simulink model "test_Dynamics_coupled_MandC"  (R2021b)
settings: Solver=ode4  StartTime=0.0  StopTime=0.01  FixedStep=0.01  RelTol=1e-3  EnableMultiTasking=on
InitFcn:
  | % ************** Initiate forces
  | % f0=[0;0;0;0;0;0];
  | % f0=[0;0;0;0;0;0;0];
  | %f_0=[0;0;0];
  | f_m=[0;1];
  | f_e=[0;0;0;0;0;0];
  | % ************** Initiate states
  | q_m=[0;0];
  | %q_dot_m=[0;0];
  | P=[0;0;0];
  | V_I0=[0;0;0];
  | % ************** Load main
  | %run(Main.m)
StopFcn:
  | format long
  | qddot=out.qddot.data(:,1)
  | qddot_ref=out.qddot_ref.data(1,:)
values from neighbouring files (symbols this model uses):
  diag_M = diagonalize(M_frak0, M_frak)    [Create_Robot.m]    (also in Main.m; diagonalize.m = zeros(6*(n+1),6*(n+1)); test_C_Main.m)
  f_0 = [0;0;0]    [Create_Robot.m]    (also in Main.m = [0;0;0;0;0;0]; test_C_Main.m)
  I0 = eye(3)*416.667    [Create_Robot.m]    (also in Main.m; test_C_Main.m)
  iota0 = [1 0 0; 0 1 0;zeros(3,3);0 0 1]    [Create_Robot.m]    (also in Main.m = eye(6,6); test_C_Main.m)
  m0 = 100    [Create_Robot.m]    (also in Main.m = 10; test_C_Main.m)
  mm = [2 2]    [Create_Robot.m]    (also in Main.m; test_C_Main.m)
  out = sim('test_Dynamics_coupled_full',0.01)    [Main.m]
  q_dot_m = [0;0]    [Create_Robot.m]    (also in Main.m; test_C_Main.m)
  X = [0 -x(3) x(2) ; x(3) 0 -x(1) ; -x(2) x(1) 0 ]    [skewsym.m]
  Xi_m_matrix = zeros(6*n,n)    [Create_Robot.m]    (also in Main.m; test_C_Main.m)
undefined symbols (not defined in the file or in its folder): Xi_m, Y, Z
libraries: sm_lib x11, nesl_utility x9
(part 1 of 2)
settings Model: Creator=Bmmog  LastModifiedBy=Bmmog
settings SimscapeCC: SimscapeLogType=all  SimscapeLogSimulationStatistics=on

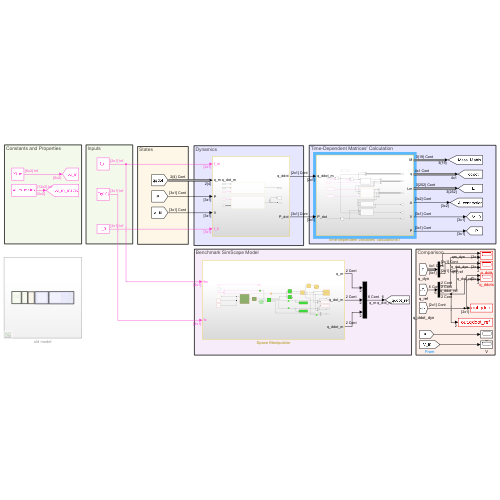
[thumbnail: Simulink's stored preview of the top-level diagram]
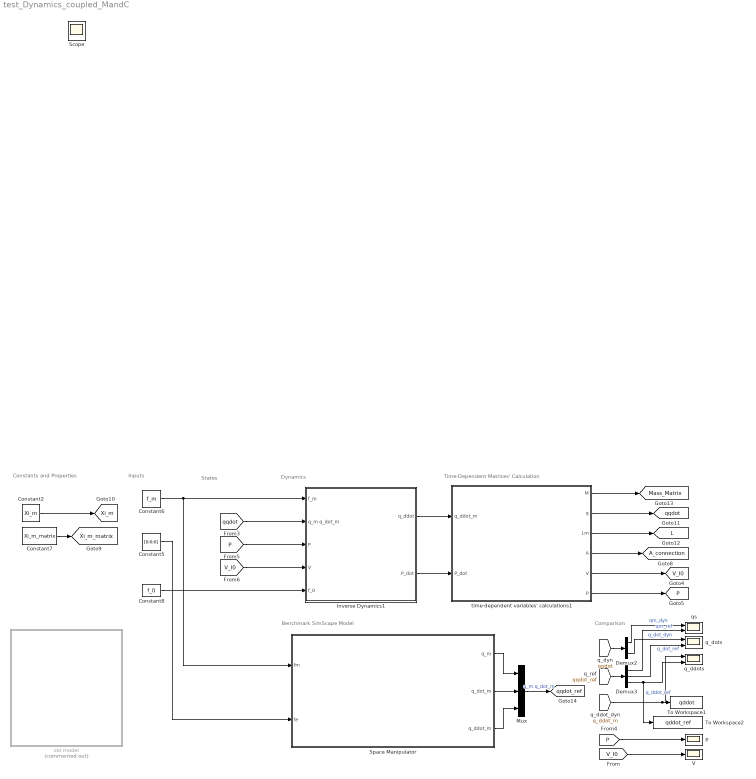
== system test_Dynamics_coupled_MandC ==
  note: States
  note: Constants and Properties
  note: Benchmark SimScape Model
  note: Comparison
  note: Inputs
  note: Dynamics
  note: Time-Dependent Matrices' Calculation
  Constant2 : Constant  Value=Xi_m  VectorParams1D=off
  Constant5 : Constant  Value=[0;0;0]  VectorParams1D=off
  Constant6 : Constant  Value=f_m  VectorParams1D=off
  Constant7 : Constant  Value=Xi_m_matrix  VectorParams1D=off
  Constant8 : Constant  Value=f_0  VectorParams1D=off
  Demux2 : Demux  Outputs=2
  Demux3 : Demux  Outputs=3
  Inverse Dynamics1 : Subsystem
  Mux : Mux  Inputs=3
  P : Scope
  Space Manipulator : Subsystem
  To Workspace1 : ToWorkspace  VariableName=qddot  SaveFormat=Timeseries  SampleTime=-1
  To Workspace2 : ToWorkspace  VariableName=qddot_ref  SaveFormat=Timeseries  SampleTime=-1
  V : Scope
  old model : Subsystem  Commented=on
  q_ddots : Scope  NumInputPorts=2
  q_dots : Scope  NumInputPorts=2
  qs : Scope  NumInputPorts=2
  time-dependent variables' calculations1 : Subsystem
  Scope : Scope
  tag scope: A_connection=global, L=global, Mass_Matrix=global, P=global, V_I0=global, Xi_m=global, Xi_m_matrix=global, qqdot=global, qqdot_ref=global
  wires:
  [V_I0] -> Inverse Dynamics1/4(V)
  Demux2/2 -> q_dots/1  "q_dot_dyn"
  Mux/1 -> [qqdot_ref]  "q_m q_dot_m"
  Space Manipulator/1(q_m) -> Mux/1
  [qqdot] -> Inverse Dynamics1/2(q_m q_dot_m)
  [q_ddot_m] -> q_ddots/1, To Workspace1/1
  Space Manipulator/2(q_dot_m) -> Mux/2
  Constant6/1 -> Space Manipulator/1(fm), Inverse Dynamics1/1(f_m)
  time-dependent variables' calculations1/1(M) -> [Mass_Matrix]
  Constant2/1 -> [Xi_m]
  [qqdot_ref] -> Demux3/1
  Demux3/1 -> qs/2  "qm_ref"
  [qqdot] -> Demux2/1
  Inverse Dynamics1/1(q_ddot) -> time-dependent variables' calculations1/1(q_ddot_m)
  Demux2/1 -> qs/1  "qm_dyn"
  Constant7/1 -> [Xi_m_matrix]
  Constant5/1 -> Space Manipulator/2(fe)
  Demux3/2 -> q_dots/2  "q_dot_ref"
  time-dependent variables' calculations1/2(q) -> [qqdot]
  Space Manipulator/3(q_ddot_m) -> Mux/3
  [P] -> Inverse Dynamics1/3(P)
  Constant8/1 -> Inverse Dynamics1/5(f_0)
  time-dependent variables' calculations1/6(P) -> [P]
  Inverse Dynamics1/2(P_dot) -> time-dependent variables' calculations1/2(P_dot)
  time-dependent variables' calculations1/3(Lm) -> [L]
  Demux3/3 -> To Workspace2/1, q_ddots/2  "q_ddot_ref"
  time-dependent variables' calculations1/5(V) -> [V_I0]
  time-dependent variables' calculations1/4(A) -> [A_connection]
  [P] -> P/1
  [V_I0] -> V/1

== system test_Dynamics_coupled_MandC/Inverse Dynamics1 ==
  f_m : Inport
  q_m q_dot_m : Inport  Port=2
  P : Inport  Port=3
  V : Inport  Port=4
  f_0 : Inport  Port=5
  Euler Poincare : Subsystem
  Internal Dynamics : Subsystem
  q_ddot : Outport
  P_dot : Outport  Port=2
  tag scope: q_ddot_m=global
  wires:
  f_m/1 -> Internal Dynamics/1(f_m)
  q_m q_dot_m/1 -> Internal Dynamics/2(q_m q_dot_m)
  Internal Dynamics/1(q_ddot) -> [q_ddot_m], q_ddot/1  "q_ddot"
  Euler Poincare/1(P_dot) -> P_dot/1  "P_dot"
  f_0/1 -> Euler Poincare/3(f_0)
  P/1 -> Euler Poincare/1(P)
  V/1 -> Euler Poincare/2(V)

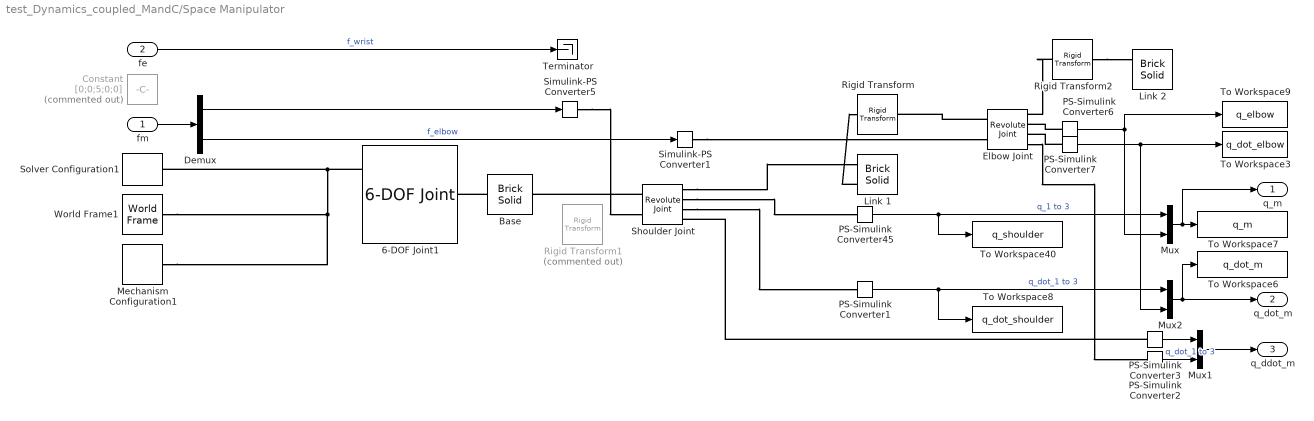
== system test_Dynamics_coupled_MandC/Space Manipulator ==
  fm : Inport
  fe : Inport  Port=2
  6-DOF Joint1 : sm_lib/Joints/6-DOF Joint  JointMode=Normal  SenseConstraintForce=off  SenseConstraintForceX=off  SenseConstraintForceY=off  SenseConstraintForceZ=off  SenseConstraintTorque=off  SenseConstraintTorqueX=off  SenseConstraintTorqueY=off  SenseConstraintTorqueZ=off  SenseTotalForce=off  SenseTotalForceX=off  SenseTotalForceY=off  SenseTotalForceZ=off  SenseTotalTorque=off  SenseTotalTorqueX=off  SenseTotalTorqueY=off  SenseTotalTorqueZ=off  CompositeWrenchDir=FollowerOnBase  CompositeWrenchFrame=BaseFrame  PxEquilibriumPosition=0  PxEquilibriumPositionUnits=m  PxSpringStiffness=0  PxSpringStiffnessUnits=N/m  PxDampingCoefficient=0  PxDampingCoefficientUnits=N/(m/s)  PxTorqueActuationMode=InputTorque  PxMotionActuationMode=ComputedMotion  PxSensePosition=off  PxSenseVelocity=off  PxSenseAcceleration=off  PxSenseTorqueForce=off  PxSenseLowerLimitTorqueForce=off  PxSenseUpperLimitTorqueForce=off  PxLowerLimitSpecify=off  PxLowerLimitBound=-1  PxLowerLimitBoundUnits=m  PxLowerLimitStiffness=1e6  PxLowerLimitStiffnessUnits=N/m  PxLowerLimitDamping=1e3  PxLowerLimitDampingUnits=N/(m/s)  PxLowerLimitTransitionRegionWidth=1e-4  PxLowerLimitTransitionRegionWidthUnits=m  PxUpperLimitSpecify=off  PxUpperLimitBound=1  PxUpperLimitBoundUnits=m  PxUpperLimitStiffness=1e6  PxUpperLimitStiffnessUnits=N/m  PxUpperLimitDamping=1e3  PxUpperLimitDampingUnits=N/(m/s)  PxUpperLimitTransitionRegionWidth=1e-4  PxUpperLimitTransitionRegionWidthUnits=m  PxPositionTargetSpecify=on  PxPositionTargetPriority=High  PxPositionTargetValue=0  PxPositionTargetValueUnits=m  PxVelocityTargetSpecify=off  PxVelocityTargetPriority=High  PxVelocityTargetValue=0  PxVelocityTargetValueUnits=m/s  PyEquilibriumPosition=0  PyEquilibriumPositionUnits=m  PySpringStiffness=0  PySpringStiffnessUnits=N/m  PyDampingCoefficient=0  PyDampingCoefficientUnits=N/(m/s)  PyTorqueActuationMode=NoTorque  PyMotionActuationMode=ComputedMotion  PySensePosition=off  PySenseVelocity=off  PySenseAcceleration=off  PySenseTorqueForce=off  PySenseLowerLimitTorqueForce=off  PySenseUpperLimitTorqueForce=off  PyLowerLimitSpecify=off  PyLowerLimitBound=-1  PyLowerLimitBoundUnits=m  PyLowerLimitStiffness=1e6  PyLowerLimitStiffnessUnits=N/m  PyLowerLimitDamping=1e3  PyLowerLimitDampingUnits=N/(m/s)  PyLowerLimitTransitionRegionWidth=1e-4  PyLowerLimitTransitionRegionWidthUnits=m  PyUpperLimitSpecify=off  PyUpperLimitBound=1  PyUpperLimitBoundUnits=m  PyUpperLimitStiffness=1e6  PyUpperLimitStiffnessUnits=N/m  PyUpperLimitDamping=1e3  PyUpperLimitDampingUnits=N/(m/s)  PyUpperLimitTransitionRegionWidth=1e-4  PyUpperLimitTransitionRegionWidthUnits=m  PyPositionTargetSpecify=on  PyPositionTargetPriority=High  PyPositionTargetValue=0  PyPositionTargetValueUnits=m  PyVelocityTargetSpecify=off  PyVelocityTargetPriority=High  PyVelocityTargetValue=0  PyVelocityTargetValueUnits=m/s  PzEquilibriumPosition=0  PzEquilibriumPositionUnits=m  PzSpringStiffness=0  PzSpringStiffnessUnits=N/m  PzDampingCoefficient=0  PzDampingCoefficientUnits=N/(m/s)  PzTorqueActuationMode=NoTorque  PzMotionActuationMode=ComputedMotion  PzSensePosition=off  PzSenseVelocity=off  PzSenseAcceleration=off  PzSenseTorqueForce=off  PzSenseLowerLimitTorqueForce=off  PzSenseUpperLimitTorqueForce=off  PzLowerLimitSpecify=off  PzLowerLimitBound=-1  PzLowerLimitBoundUnits=m  PzLowerLimitStiffness=1e6  PzLowerLimitStiffnessUnits=N/m  PzLowerLimitDamping=1e3  PzLowerLimitDampingUnits=N/(m/s)  PzLowerLimitTransitionRegionWidth=1e-4  PzLowerLimitTransitionRegionWidthUnits=m  PzUpperLimitSpecify=off  PzUpperLimitBound=1  PzUpperLimitBoundUnits=m  PzUpperLimitStiffness=1e6  PzUpperLimitStiffnessUnits=N/m  PzUpperLimitDamping=1e3  PzUpperLimitDampingUnits=N/(m/s)  PzUpperLimitTransitionRegionWidth=1e-4  PzUpperLimitTransitionRegionWidthUnits=m  PzPositionTargetSpecify=on  PzPositionTargetPriority=High  PzPositionTargetValue=0  PzPositionTargetValueUnits=m  PzVelocityTargetSpecify=off  PzVelocityTargetPriority=High  PzVelocityTargetValue=0  PzVelocityTargetValueUnits=m/s  SphDefPosRotationMethod=None  SphDefPosRotationAngleUnits=deg  SphDefPosRotationStandardAxis=+Z  SphDefPosRotationAngle=0.0  SphDefPosRotationArbitraryAxis=[0 0 1]  SphDefPosFollAlignAxisA=+X  SphDefPosBaseAlignAxisA=+Y  SphDefPosFollAlignAxisB=+Y  SphDefPosBaseAlignAxisB=+Z  SphDefPosRotationSequenceAxes=FollowerAxes  SphDefPosRotationSequence=XYX  SphDefPosRotationSequenceAngles=[0 0 0]  SphDefPosRotationSequenceAnglesUnits=deg  SphDefPosRotationMatrix=[1 0 0; 0 1 0; 0 0 1]  SphEqPosRotationMethod=None  SphEqPosRotationAngleUnits=deg  SphEqPosRotationStandardAxis=+Z  SphEqPosRotationAngle=0.0  SphEqPosRotationArbitraryAxis=[0 0 1]  SphEqPosFollAlignAxisA=+X  SphEqPosBaseAlignAxisA=+Y  SphEqPosFollAlignAxisB=+Y  SphEqPosBaseAlignAxisB=+Z  SphEqPosRotationSequenceAxes=FollowerAxes  SphEqPosRotationSequence=XYX  SphEqPosRotationSequenceAngles=[0 0 0]  SphEqPosRotationSequenceAnglesUnits=deg  SphEqPosRotationMatrix=[1 0 0; 0 1 0; 0 0 1]  SphSpringStiffness=0  SphSpringStiffnessUnits=N*m/deg  SphDampingCoefficient=0  SphDampingCoefficientUnits=N*m/(deg/s)  SphActuateTorqueX=off  SphActuateTorqueY=off  SphActuateTorqueZ=off  SphActuateTorque=off  SphTorqueActuationMode=NoTorque  SphMotionActuationMode=ComputedMotion  SphActuationFrame=BaseFrame  SphSensePosition=off  SphSenseVelocityX=off  SphSenseVelocityY=off  SphSenseVelocityZ=off  SphSenseVelocity=off  SphSenseAccelerationX=off  SphSenseAccelerationY=off  SphSenseAccelerationZ=off  SphSenseAcceleration=off  SphSenseTorqueX=off  SphSenseTorqueY=off  SphSenseTorqueZ=off  SphSenseTorqueForce=off  SphSenseLowerLimitTorqueMag=off  SphSenseUpperLimitTorqueMag=off  SphSensingFrame=BaseFrame  SphLowerLimitSpecify=off  SphLowerLimitBound=15  SphLowerLimitBoundUnits=deg  SphLowerLimitStiffness=1e4  SphLowerLimitStiffnessUnits=N*m/deg  SphLowerLimitDamping=10  SphLowerLimitDampingUnits=N*m/(deg/s)  SphLowerLimitTransitionRegionWidth=0.1  SphLowerLimitTransitionRegionWidthUnits=deg  SphUpperLimitSpecify=off  SphUpperLimitBound=45  SphUpperLimitBoundUnits=deg  SphUpperLimitStiffness=1e4  SphUpperLimitStiffnessUnits=N*m/deg  SphUpperLimitDamping=10  SphUpperLimitDampingUnits=N*m/(deg/s)  SphUpperLimitTransitionRegionWidth=0.1  SphUpperLimitTransitionRegionWidthUnits=deg  SphPositionTargetRotationMethod=RotationSequence  SphPositionTargetRotationAngleUnits=deg  SphPositionTargetRotationStandardAxis=+Z  SphPositionTargetRotationAngle=0.0  SphPositionTargetRotationArbitraryAxis=[0 0 1]  SphPositionTargetFollAlignAxisA=+X  SphPositionTargetBaseAlignAxisA=+Y  SphPositionTargetFollAlignAxisB=+Y  SphPositionTargetBaseAlignAxisB=+Z  SphPositionTargetRotationSequenceAxes=FollowerAxes  SphPositionTargetRotationSequence=ZYX  SphPositionTargetRotationSequenceAngles=[0 0 0]  SphPositionTargetRotationSequenceAnglesUnits=deg  SphPositionTargetRotationMatrix=[1 0 0; 0 1 0; 0 0 1]  SphPositionTargetSpecify=off  SphPositionTargetPriority=High  SphVelocityTargetValue=[0 0.5 0.5]  SphVelocityTargetValueUnits=rad/s  SphVelocityTargetSpecify=off  SphVelocityTargetPriority=High  SphVelocityTargetInFollowerFrame=on
  Base : sm_lib/Body Elements/Brick Solid  GraphicAmbientColor=[0.15 0.15 0.15 1.0]  BasedOnType=Mass  BrickDimensions=[5, 5, 5]  BrickDimensionUnits=m  CenterOfMass=[0 0 0]  CenterOfMassUnits=m  GraphicDiffuseColor=[0.5 0.5 0.5]  Density=1000  DensityUnits=kg/m^3  DoExposeReferenceFrame=on  GraphicEmissiveColor=[0.0 0.0 0.0 1.0]  ExportEntireGeometry=off  SerializedFrames=<Frames><Frame><Id>Frame1</Id><Value><Name>F1</Name><Origin><Source>GeometricFeature</Source><FeatureName>+z surface</FeatureName></Origin><PrimaryAxis><DefinedDirection>+X</DefinedDirection><Source>ReferenceFrame</Source><SourceDirection>+Z</SourceDirection><FeatureName></FeatureName></PrimaryAxis><SecondaryAxis><DefinedDirection>+Z</DefinedDirection><Source>ReferenceFrame</Source><SourceDirection>+X</SourceDirection><FeatureName></FeatureName></SecondaryAxis></Value></Frame></Frames>  MarkerShape=Sphere  MarkerSize=10  GraphicType=FromGeometry  InertiaType=Custom  Mass=m0  MassUnits=kg  MomentsOfInertia=[I0(1,1) I0(2,2) I0(3,3)]  MomentsOfInertiaUnits=kg*m^2  GraphicOpacity=1.0  ProductsOfInertia=[0 0 0]  ProductsOfInertiaUnits=kg*m^2  GraphicShininess=75  GraphicSpecularColor=[0.5 0.5 0.5 1.0]  GraphicVisPropType=SimpleVisualProperties
  Constant : Constant  Commented=on  Value=[0;0;5;0;0]
  Demux : Demux  Outputs=2
  Elbow Joint : sm_lib/Joints/Revolute Joint  JointMode=Normal  SenseConstraintForce=off  SenseConstraintForceX=off  SenseConstraintForceY=off  SenseConstraintForceZ=off  SenseConstraintTorque=off  SenseConstraintTorqueX=off  SenseConstraintTorqueY=off  SenseConstraintTorqueZ=off  SenseTotalForce=off  SenseTotalForceX=off  SenseTotalForceY=off  SenseTotalForceZ=off  SenseTotalTorque=off  SenseTotalTorqueX=off  SenseTotalTorqueY=off  SenseTotalTorqueZ=off  CompositeWrenchDir=FollowerOnBase  CompositeWrenchFrame=BaseFrame  EquilibriumPosition=0  EquilibriumPositionUnits=rad  SpringStiffness=0  SpringStiffnessUnits=N*m/rad  DampingCoefficient=0  DampingCoefficientUnits=N*m/(rad/s)  TorqueActuationMode=InputTorque  MotionActuationMode=ComputedMotion  SensePosition=on  SenseVelocity=on  SenseAcceleration=on  SenseTorqueForce=off  SenseLowerLimitTorqueForce=off  SenseUpperLimitTorqueForce=off  LowerLimitSpecify=off  LowerLimitBound=-90  LowerLimitBoundUnits=deg  LowerLimitStiffness=1e4  LowerLimitStiffnessUnits=N*m/deg  LowerLimitDamping=10  LowerLimitDampingUnits=N*m/(deg/s)  LowerLimitTransitionRegionWidth=0.1  LowerLimitTransitionRegionWidthUnits=deg  UpperLimitSpecify=off  UpperLimitBound=90  UpperLimitBoundUnits=deg  UpperLimitStiffness=1e4  UpperLimitStiffnessUnits=N*m/deg  UpperLimitDamping=10  UpperLimitDampingUnits=N*m/(deg/s)  UpperLimitTransitionRegionWidth=0.1  UpperLimitTransitionRegionWidthUnits=deg  PositionTargetSpecify=on  PositionTargetPriority=High  PositionTargetValue=q_m(2)  PositionTargetValueUnits=rad  VelocityTargetSpecify=on  VelocityTargetPriority=High  VelocityTargetValue=q_dot_m(2)  VelocityTargetValueUnits=rad/s
  "Link 1 " : sm_lib/Body Elements/Brick Solid  GraphicAmbientColor=[0.15 0.15 0.15 1.0]  BasedOnType=Mass  BrickDimensions=[0.1, 0.1, 4.5]  BrickDimensionUnits=m  CenterOfMass=[0 0 0]  CenterOfMassUnits=m  GraphicDiffuseColor=[0.5 0.5 0.5]  Density=1000  DensityUnits=kg/m^3  DoExposeReferenceFrame=on  GraphicEmissiveColor=[0.0 0.0 0.0 1.0]  ExportEntireGeometry=off  SerializedFrames=<Frames><Frame><Id>Frame1</Id><Value><Name>F1</Name><Origin><Source>GeometricFeature</Source><FeatureName>-z surface</FeatureName></Origin><PrimaryAxis><DefinedDirection>+X</DefinedDirection><Source>ReferenceFrame</Source><SourceDirection>+Z</SourceDirection><FeatureName></FeatureName></PrimaryAxis><SecondaryAxis><DefinedDirection>+Z</DefinedDirection><Source>ReferenceFrame</Source><SourceDirection>+X</SourceDirection><FeatureName></FeatureName></SecondaryAxis></Value></Frame><Frame><Id>Frame2</Id><Value><Name>F2</Name><Origin><Source>GeometricFeature</Source><FeatureName>+z surface</FeatureName></Origin><PrimaryAxis><DefinedDirection>+X</DefinedDirection><Source>ReferenceFrame</Source><SourceDirection>+Z</SourceDirection><FeatureName></FeatureName></PrimaryAxis><SecondaryAxis><DefinedDirection>+Z</DefinedDirection><Source>ReferenceFrame</Source><SourceDirection>+X</SourceDirection><FeatureName></FeatureName></SecondaryAxis></Value></Frame></Frames>  MarkerShape=Sphere  MarkerSize=10  GraphicType=FromGeometry  InertiaType=Custom  Mass=mm(1)  MassUnits=kg  MomentsOfInertia=[3.37667 3.37667 0.00333333]  MomentsOfInertiaUnits=kg*m^2  GraphicOpacity=1.0  ProductsOfInertia=[0 0 0]  ProductsOfInertiaUnits=kg*m^2  GraphicShininess=75  GraphicSpecularColor=[0.5 0.5 0.5 1.0]  GraphicVisPropType=SimpleVisualProperties
  Link 2 : sm_lib/Body Elements/Brick Solid  GraphicAmbientColor=[0.15 0.15 0.15 1.0]  BasedOnType=Mass  BrickDimensions=[0.1, 0.1,4.5]  BrickDimensionUnits=m  CenterOfMass=[0 0 0]  CenterOfMassUnits=m  GraphicDiffuseColor=[0.5 0.5 0.5]  Density=1000  DensityUnits=kg/m^3  DoExposeReferenceFrame=on  GraphicEmissiveColor=[0.0 0.0 0.0 1.0]  ExportEntireGeometry=off  SerializedFrames=<Frames><Frame><Id>Frame1</Id><Value><Name>F1</Name><Origin><Source>GeometricFeature</Source><FeatureName>-z surface</FeatureName></Origin><PrimaryAxis><DefinedDirection>+X</DefinedDirection><Source>ReferenceFrame</Source><SourceDirection>+Z</SourceDirection><FeatureName></FeatureName></PrimaryAxis><SecondaryAxis><DefinedDirection>+Z</DefinedDirection><Source>ReferenceFrame</Source><SourceDirection>+Y</SourceDirection><FeatureName></FeatureName></SecondaryAxis></Value></Frame><Frame><Id>Frame2</Id><Value><Name>F2</Name><Origin><Source>GeometricFeature</Source><FeatureName>+z surface</FeatureName></Origin><PrimaryAxis><DefinedDirection>+X</DefinedDirection><Source>ReferenceFrame</Source><SourceDirection>+Z</SourceDirection><FeatureName></FeatureName></PrimaryAxis><SecondaryAxis><DefinedDirection>+Z</DefinedDirection><Source>ReferenceFrame</Source><SourceDirection>+Y</SourceDirection><FeatureName></FeatureName></SecondaryAxis></Value></Frame></Frames>  MarkerShape=Sphere  MarkerSize=10  GraphicType=FromGeometry  InertiaType=Custom  Mass=mm(2)  MassUnits=kg  MomentsOfInertia=[3.37667 3.37667 0.00333333]  MomentsOfInertiaUnits=kg*m^2  GraphicOpacity=1.0  ProductsOfInertia=[0 0 0]  ProductsOfInertiaUnits=kg*m^2  GraphicShininess=75  GraphicSpecularColor=[0.5 0.5 0.5 1.0]  GraphicVisPropType=SimpleVisualProperties
  Mechanism Configuration1 : sm_lib/Utilities/Mechanism Configuration  UniformGravity=Constant  GravityVector=[0 0 0]  GravityUnits=m/s^2  LinearizationDelta=0.001  JointModeTransitionNonlinearIterations=2
  Mux : Mux  Inputs=2
  Mux1 : Mux  Inputs=2
  Mux2 : Mux  Inputs=2
  PS-Simulink Converter{1..3,6..7,45} (6 alike) : nesl_utility/PS-Simulink Converter  PhysicalDomain=network_engine_domain  SubClassName=ps_output  LeftPortType=input  RightPortType=output  PseudoPeriodic=off  Frequencies=[]  Unit=inherit  AffineConversion=off
      settings: SourceProductBaseCode=PW,SS
  Rigid Transform : sm_lib/Frames and Transforms/Rigid Transform  TranslationMethod=None  TranslationStandardOffset=0  TranslationLengthUnit=m  TranslationStandardAxis=+Z  TranslationCartesianOffset=[0 0 0]  TranslationROffset=0  TranslationROffsetUnits=m  TranslationZOffset=0  TranslationZOffsetUnits=m  TranslationThetaOffset=0  TranslationThetaOffsetUnits=deg  RotationMethod=StandardAxis  RotationAngleUnits=deg  RotationStandardAxis=+X  RotationAngle=90  RotationArbitraryAxis=[0 0 1]  FollAlignAxisA=+X  BaseAlignAxisA=+Y  FollAlignAxisB=+Y  BaseAlignAxisB=+Z  RotationSequenceAxes=FollowerAxes  RotationSequence=XYX  RotationSequenceAngles=[0 0 0]  RotationSequenceAnglesUnits=deg  RotationMatrix=[1 0 0; 0 1 0; 0 0 1]
  Rigid Transform1 : sm_lib/Frames and Transforms/Rigid Transform  Commented=on  TranslationMethod=Cartesian  TranslationStandardOffset=0  TranslationLengthUnit=m  TranslationStandardAxis=+Z  TranslationCartesianOffset=[0 0 2.5]  TranslationROffset=0  TranslationROffsetUnits=m  TranslationZOffset=0  TranslationZOffsetUnits=m  TranslationThetaOffset=0  TranslationThetaOffsetUnits=deg  RotationMethod=RotationMatrix  RotationAngleUnits=deg  RotationStandardAxis=+X  RotationAngle=90  RotationArbitraryAxis=[0 0 1]  FollAlignAxisA=+X  BaseAlignAxisA=+Y  FollAlignAxisB=+Y  BaseAlignAxisB=+Z  RotationSequenceAxes=FollowerAxes  RotationSequence=XYX  RotationSequenceAngles=[0 0 0]  RotationSequenceAnglesUnits=deg  RotationMatrix=[0 0 1; 0 -1 0; 1 0 0]
  Rigid Transform2 : sm_lib/Frames and Transforms/Rigid Transform  TranslationMethod=None  TranslationStandardOffset=0  TranslationLengthUnit=m  TranslationStandardAxis=+Z  TranslationCartesianOffset=[0 0 0]  TranslationROffset=0  TranslationROffsetUnits=m  TranslationZOffset=0  TranslationZOffsetUnits=m  TranslationThetaOffset=0  TranslationThetaOffsetUnits=deg  RotationMethod=None  RotationAngleUnits=deg  RotationStandardAxis=+Y  RotationAngle=0  RotationArbitraryAxis=[0 0 1]  FollAlignAxisA=+X  BaseAlignAxisA=+Y  FollAlignAxisB=+Y  BaseAlignAxisB=+Z  RotationSequenceAxes=FollowerAxes  RotationSequence=XYX  RotationSequenceAngles=[0 0 0]  RotationSequenceAnglesUnits=deg  RotationMatrix=[1 0 0; 0 1 0; 0 0 1]
  Shoulder Joint : sm_lib/Joints/Revolute Joint  JointMode=Normal  SenseConstraintForce=off  SenseConstraintForceX=off  SenseConstraintForceY=off  SenseConstraintForceZ=off  SenseConstraintTorque=off  SenseConstraintTorqueX=off  SenseConstraintTorqueY=off  SenseConstraintTorqueZ=off  SenseTotalForce=off  SenseTotalForceX=off  SenseTotalForceY=off  SenseTotalForceZ=off  SenseTotalTorque=off  SenseTotalTorqueX=off  SenseTotalTorqueY=off  SenseTotalTorqueZ=off  CompositeWrenchDir=FollowerOnBase  CompositeWrenchFrame=BaseFrame  EquilibriumPosition=0  EquilibriumPositionUnits=rad  SpringStiffness=0  SpringStiffnessUnits=N*m/rad  DampingCoefficient=0  DampingCoefficientUnits=N*m/(rad/s)  TorqueActuationMode=InputTorque  MotionActuationMode=ComputedMotion  SensePosition=on  SenseVelocity=on  SenseAcceleration=on  SenseTorqueForce=off  SenseLowerLimitTorqueForce=off  SenseUpperLimitTorqueForce=off  LowerLimitSpecify=off  LowerLimitBound=-90  LowerLimitBoundUnits=deg  LowerLimitStiffness=1e4  LowerLimitStiffnessUnits=N*m/deg  LowerLimitDamping=10  LowerLimitDampingUnits=N*m/(deg/s)  LowerLimitTransitionRegionWidth=0.1  LowerLimitTransitionRegionWidthUnits=deg  UpperLimitSpecify=off  UpperLimitBound=90  UpperLimitBoundUnits=deg  UpperLimitStiffness=1e4  UpperLimitStiffnessUnits=N*m/deg  UpperLimitDamping=10  UpperLimitDampingUnits=N*m/(deg/s)  UpperLimitTransitionRegionWidth=0.1  UpperLimitTransitionRegionWidthUnits=deg  PositionTargetSpecify=on  PositionTargetPriority=High  PositionTargetValue=q_m(1)  PositionTargetValueUnits=rad  VelocityTargetSpecify=on  VelocityTargetPriority=High  VelocityTargetValue=q_dot_m(1)  VelocityTargetValueUnits=rad/s
  Simulink-PS Converter1 : nesl_utility/Simulink-PS Converter  PhysicalDomain=network_engine_domain  SubClassName=ps_input  LeftPortType=input  RightPortType=output  PseudoPeriodic=off  Frequencies=[]  NoiseDistribution=none  NoiseParameters=[]  Unit=1  AffineConversion=off  FilteringAndDerivatives=provide  SimscapeFilterOrder=1  InputFilterTimeConstant=0.001  UdotUserProvided=0
      settings: SourceProductBaseCode=PW,SS
  Simulink-PS Converter5 : nesl_utility/Simulink-PS Converter  PhysicalDomain=network_engine_domain  SubClassName=ps_input  LeftPortType=input  RightPortType=output  PseudoPeriodic=off  Frequencies=[]  NoiseDistribution=none  NoiseParameters=[]  Unit=1  AffineConversion=off  FilteringAndDerivatives=provide  SimscapeFilterOrder=1  InputFilterTimeConstant=0.001  UdotUserProvided=0
      settings: SourceProductBaseCode=PW,SS
  Solver Configuration1 : nesl_utility/Solver Configuration  PhysicalDomain=network_engine_domain  SubClassName=solver  LeftPortType=input  RightPortType=generic  Tones=[]  Harmonics=[]  SimulateNoise=off  Profile=off  UseLocalSampling=off  EnableSwitchedLinearOptims=on  FrequencyDomain=off  UseCCode=off  RelTol=0.001  AbsTol=1e-06  MinStep=1e-09  ToWorkspace=off  RevertToSquareIcSolve=off  NumHomotopyIterations=100  PhasorMode=off  PhasorModeNumHarmonics=1  DoDC=off  ResidualTolerance=1e-09  UseLocalSolver=off  LocalSolverChoice=NE_BACKWARD_EULER_ADVANCER  LocalSolverSampleTime=0.001  DoFixedCost=off  MaxNonlinIter=3  MaxModeIter=2  ComputeImpulses=off  ImpulseIterations=2  LinearAlgebra=Sparse  EquationFormulation=NE_TIME_EF  DelaysMemoryBudget=1024  AutomaticFiltering=on  FilteringTimeConstant=0.001  PartitionStorageMethod=AS_NEEDED  PartitionMemoryBudget=1024  PartitionMethod=FAST
      settings: SourceProductBaseCode=PW,SS
  Terminator : Terminator
  To Workspace3 : ToWorkspace  VariableName=q_dot_elbow  SampleTime=-1
  To Workspace40 : ToWorkspace  VariableName=q_shoulder  SampleTime=-1
  To Workspace6 : ToWorkspace  VariableName=q_dot_m  SampleTime=-1
  To Workspace7 : ToWorkspace  VariableName=q_m  SampleTime=-1
  To Workspace8 : ToWorkspace  VariableName=q_dot_shoulder  SampleTime=-1
  To Workspace9 : ToWorkspace  VariableName=q_elbow  SampleTime=-1
  World Frame1 : sm_lib/Frames and Transforms/World Frame
  q_m : Outport
  q_dot_m : Outport  Port=2
  q_ddot_m : Outport  Port=3
  wires:
  PS-Simulink Converter6/1 -> To Workspace9/1, Mux/2
  fm/1 -> Demux/1
  PS-Simulink Converter7/1 -> Mux2/2, To Workspace3/1
  PS-Simulink Converter45/1 -> Mux/1, To Workspace40/1  "q_1 to 3"
  Mux/1 -> q_m/1, To Workspace7/1
  Mux2/1 -> To Workspace6/1, q_dot_m/1
  Demux/2 -> Simulink-PS Converter1/1  "f_elbow"
  PS-Simulink Converter1/1 -> Mux2/1, To Workspace8/1  "q_dot_1 to 3"
  PS-Simulink Converter2/1 -> Mux1/2  "q_dot_1 to 3"
  PS-Simulink Converter3/1 -> Mux1/1
  Mux1/1 -> q_ddot_m/1
  Demux/1 -> Simulink-PS Converter5/1
  fe/1 -> Terminator/1  "f_wrist"
  connections:
  Rigid Transform2/RConn1 -- Link 2/LConn1
  Shoulder Joint/RConn1 -- "Link 1 "/LConn1
  Shoulder Joint/RConn2 -- PS-Simulink Converter45/LConn1
  Elbow Joint/LConn1 -- Rigid Transform/RConn1
  PS-Simulink Converter6/LConn1 -- Elbow Joint/RConn2
  "Link 1 "/LConn2 -- Rigid Transform/LConn1
  Rigid Transform2/LConn1 -- Elbow Joint/RConn1
  Shoulder Joint/RConn3 -- PS-Simulink Converter1/LConn1
  PS-Simulink Converter7/LConn1 -- Elbow Joint/RConn3
  Solver Configuration1/RConn1 -- Mechanism Configuration1/RConn1 -- World Frame1/RConn1 -- 6-DOF Joint1/LConn1
  Elbow Joint/RConn4 -- PS-Simulink Converter2/LConn1
  PS-Simulink Converter3/LConn1 -- Shoulder Joint/RConn4
  Shoulder Joint/LConn1 -- Base/LConn1
  Simulink-PS Converter1/RConn1 -- Elbow Joint/LConn2
  Simulink-PS Converter5/RConn1 -- Shoulder Joint/LConn2
  Base/RConn1 -- 6-DOF Joint1/RConn1

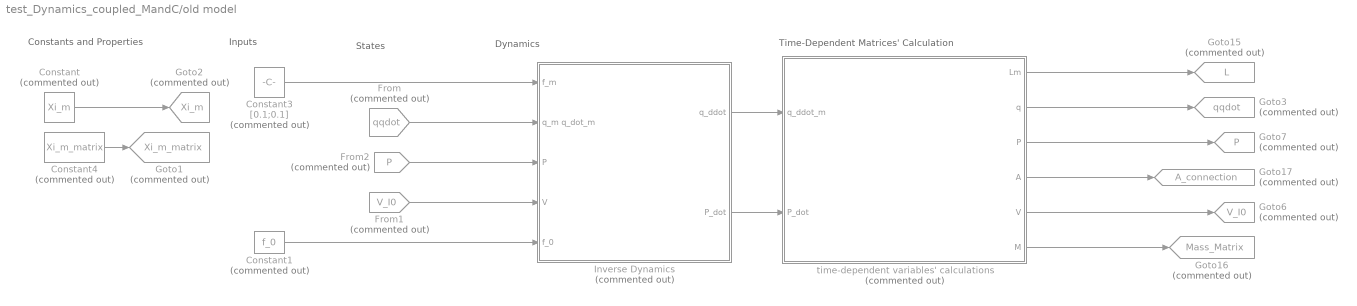
== system test_Dynamics_coupled_MandC/old model ==
  note: States
  note: Inputs
  note: Time-Dependent Matrices' Calculation
  note: Constants and Properties
  note: Dynamics
  Constant : Constant  Commented=on  Value=Xi_m  VectorParams1D=off
  Constant1 : Constant  Commented=on  Value=f_0  VectorParams1D=off
  Constant3 : Constant  Commented=on  Value=[0.1;0.1]  VectorParams1D=off
  Constant4 : Constant  Commented=on  Value=Xi_m_matrix  VectorParams1D=off
  From : From  Commented=on  GotoTag=qqdot  TagVisibility=global
  From1 : From  Commented=on  GotoTag=V_I0  TagVisibility=global
  From2 : From  Commented=on  GotoTag=P  TagVisibility=global
  Goto1 : Goto  Commented=on  GotoTag=Xi_m_matrix  TagVisibility=global
  Goto15 : Goto  Commented=on  GotoTag=L  TagVisibility=global
  Goto16 : Goto  Commented=on  GotoTag=Mass_Matrix  TagVisibility=global
  Goto17 : Goto  Commented=on  GotoTag=A_connection  TagVisibility=global
  Goto2 : Goto  Commented=on  GotoTag=Xi_m  TagVisibility=global
  Goto3 : Goto  Commented=on  GotoTag=qqdot  TagVisibility=global
  Goto6 : Goto  Commented=on  GotoTag=V_I0  TagVisibility=global
  Goto7 : Goto  Commented=on  GotoTag=P  TagVisibility=global
  Inverse Dynamics : Subsystem  Commented=on
  time-dependent variables' calculations : Subsystem  Commented=on
  wires:
  Constant3/1 -> Inverse Dynamics/1(f_m)
  From1/1 -> Inverse Dynamics/4(V)
  time-dependent variables' calculations/6(M) -> Goto16/1
  Inverse Dynamics/2(P_dot) -> time-dependent variables' calculations/2(P_dot)
  time-dependent variables' calculations/2(q) -> Goto3/1
  Constant1/1 -> Inverse Dynamics/5(f_0)
  Constant/1 -> Goto2/1
  time-dependent variables' calculations/1(Lm) -> Goto15/1
  time-dependent variables' calculations/3(P) -> Goto7/1
  From/1 -> Inverse Dynamics/2(q_m q_dot_m)
  Constant4/1 -> Goto1/1
  time-dependent variables' calculations/5(V) -> Goto6/1
  Inverse Dynamics/1(q_ddot) -> time-dependent variables' calculations/1(q_ddot_m)
  time-dependent variables' calculations/4(A) -> Goto17/1
  From2/1 -> Inverse Dynamics/3(P)

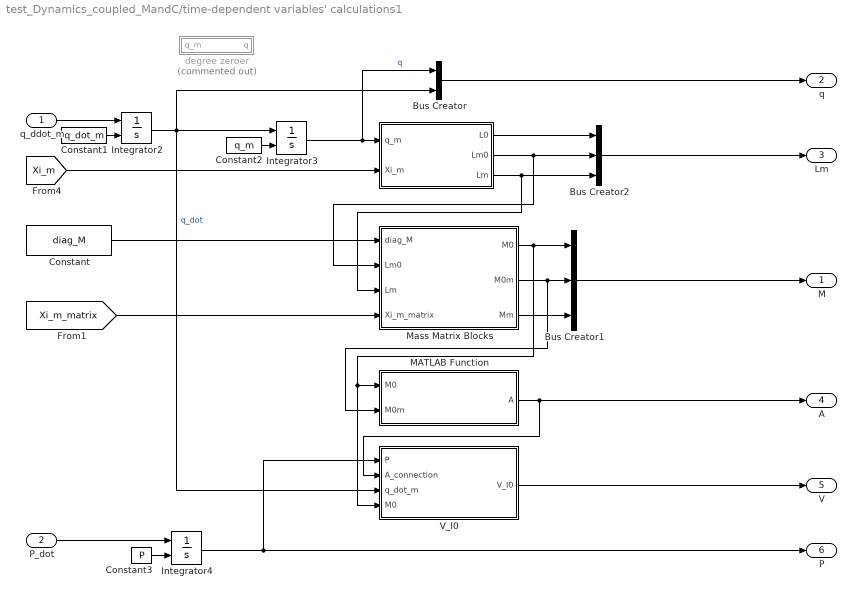
== system test_Dynamics_coupled_MandC/time-dependent variables' calculations1 ==
  q_ddot_m : Inport
  P_dot : Inport  Port=2
  " " : MATLAB Function  TreatAsAtomicUnit=on
  Bus Creator : BusCreator  Inputs=2
  Bus Creator1 : BusCreator  Inputs=3
  Bus Creator2 : BusCreator  Inputs=3
  Constant : Constant  Value=diag_M  VectorParams1D=off
  Constant1 : Constant  Value=q_dot_m  VectorParams1D=off
  Constant2 : Constant  Value=q_m  VectorParams1D=off
  Constant3 : Constant  Value=P  VectorParams1D=off
  Integrator2 : Integrator  InitialConditionSource=external  InitialCondition=q_dot_m
  Integrator3 : Integrator  InitialConditionSource=external
  Integrator4 : Integrator  InitialConditionSource=external
  MATLAB Function : MATLAB Function  TreatAsAtomicUnit=on
  Mass Matrix Blocks : Subsystem
  V_I0 : MATLAB Function  TreatAsAtomicUnit=on
  degree zeroer : MATLAB Function  Commented=on  TreatAsAtomicUnit=on
  M : Outport
  q : Outport  Port=2
  Lm : Outport  Port=3
  A : Outport  Port=4
  V : Outport  Port=5
  P : Outport  Port=6
  wires:
  Mass Matrix Blocks/3(Mm) -> Bus Creator1/3
  Integrator2/1 -> V_I0/3(q_dot_m), Bus Creator/2, Integrator3/1  "q_dot"
  q_ddot_m/1 -> Integrator2/1
  " "/1(L0) -> Bus Creator2/1
  " "/3(Lm) -> Bus Creator2/3, Mass Matrix Blocks/3(Lm)
  " "/2(Lm0) -> Bus Creator2/2, Mass Matrix Blocks/2(Lm0)
  Constant/1 -> Mass Matrix Blocks/1(diag_M)
  [Xi_m_matrix] -> Mass Matrix Blocks/4(Xi_m_matrix)
  [Xi_m] -> " "/2(Xi_m)
  Integrator3/1 -> Bus Creator/1, " "/1(q_m)  "q"
  Bus Creator/1 -> q/1
  Constant1/1 -> Integrator2/2
  Constant2/1 -> Integrator3/2
  Bus Creator2/1 -> Lm/1
  Bus Creator1/1 -> M/1
  Mass Matrix Blocks/2(M0m) -> MATLAB Function/2(M0m), Bus Creator1/2
  Mass Matrix Blocks/1(M0) -> V_I0/4(M0), MATLAB Function/1(M0), Bus Creator1/1
  MATLAB Function/1(A) -> V_I0/2(A_connection), A/1
  V_I0/1(V_I0) -> V/1
  P_dot/1 -> Integrator4/1
  Integrator4/1 -> V_I0/1(P), P/1
  Constant3/1 -> Integrator4/2

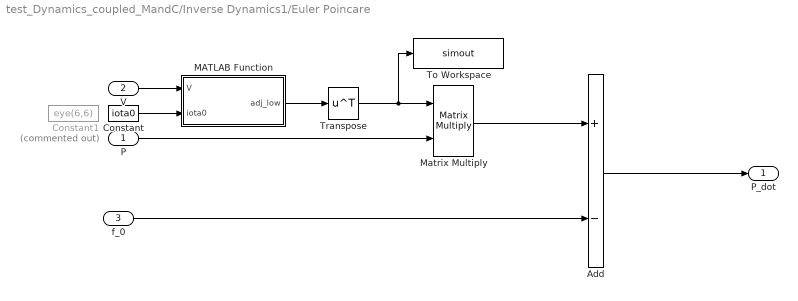
== system test_Dynamics_coupled_MandC/Inverse Dynamics1/Euler Poincare ==
  P : Inport
  V : Inport  Port=2
  f_0 : Inport  Port=3
  Add : Sum  Inputs=+-
  Constant : Constant  Value=iota0
  Constant1 : Constant  Commented=on  Value=eye(6,6)
  MATLAB Function : MATLAB Function  TreatAsAtomicUnit=on
  Matrix Multiply : Product  Multiplication=Matrix(*)
  To Workspace : ToWorkspace  VariableName=simout  SaveFormat=Timeseries  SampleTime=-1
  Transpose : Math  Operator=transpose  SaturateOnIntegerOverflow=on
  P_dot : Outport
  wires:
  P/1 -> Matrix Multiply/2
  MATLAB Function/1(adj_low) -> Transpose/1
  V/1 -> MATLAB Function/1(V)
  Transpose/1 -> To Workspace/1, Matrix Multiply/1
  Matrix Multiply/1 -> Add/1
  f_0/1 -> Add/2
  Add/1 -> P_dot/1
  Constant/1 -> MATLAB Function/2(iota0)

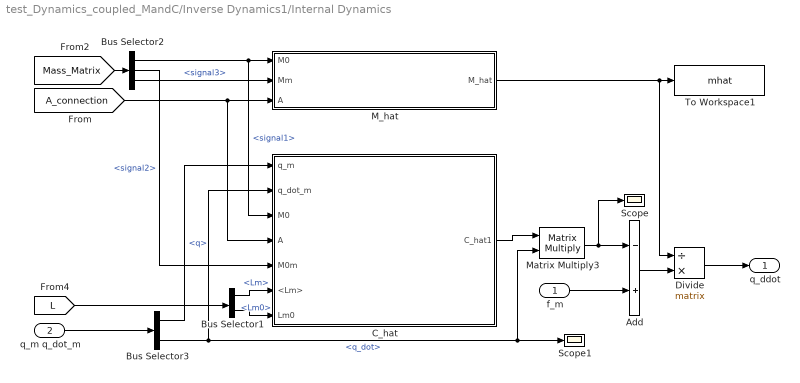
== system test_Dynamics_coupled_MandC/Inverse Dynamics1/Internal Dynamics ==
  f_m : Inport
  q_m q_dot_m : Inport  Port=2
  Add : Sum  Inputs=-+
  Bus Selector1 : BusSelector  OutputSignals=Lm,Lm0
  Bus Selector2 : BusSelector  OutputSignals=signal1,signal2,signal3
  Bus Selector3 : BusSelector  OutputSignals=q,q_dot
  C_hat : Subsystem
  Divide : Product  Inputs=/*  Multiplication=Matrix(*)
  M_hat : MATLAB Function  TreatAsAtomicUnit=on
  Matrix Multiply3 : Product  Multiplication=Matrix(*)
  Scope : Scope
  Scope1 : Scope
  To Workspace1 : ToWorkspace  VariableName=mhat  SaveFormat=Timeseries  SampleTime=-1
  q_ddot : Outport
  wires:
  Bus Selector3/1 -> C_hat/1(q_m)  "<q>"
  f_m/1 -> Add/2
  Bus Selector2/3 -> M_hat/2(Mm)  "<signal3>"
  q_m q_dot_m/1 -> Bus Selector3/1
  C_hat/1(C_hat1) -> Matrix Multiply3/1
  [A_connection] -> M_hat/3(A), C_hat/4(A)
  [L] -> Bus Selector1/1
  Bus Selector2/1 -> M_hat/1(M0), C_hat/3(M0)  "<signal1>"
  [Mass_Matrix] -> Bus Selector2/1
  Bus Selector3/2 -> C_hat/2(q_dot_m), Matrix Multiply3/2, Scope1/1  "<q_dot>"
  Divide/1 -> q_ddot/1
  Bus Selector2/2 -> C_hat/5(M0m)  "<signal2>"
  Bus Selector1/2 -> C_hat/7(Lm0)  "<Lm0>"
  Bus Selector1/1 -> C_hat/6(<Lm>)  "<Lm>"
  Matrix Multiply3/1 -> Scope/1, Add/1
  Add/1 -> Divide/2
  M_hat/1(M_hat) -> To Workspace1/1, Divide/1

== system test_Dynamics_coupled_MandC/old model/Inverse Dynamics ==
  f_m : Inport
  q_m q_dot_m : Inport  Port=2
  P : Inport  Port=3
  V : Inport  Port=4
  f_0 : Inport  Port=5
  Euler Poincare : Subsystem
  Internal Dynamics : Subsystem
  q_ddot : Outport
  P_dot : Outport  Port=2
  wires:
  f_m/1 -> Internal Dynamics/1(f_m)
  Internal Dynamics/1(q_ddot) -> q_ddot/1  "q_ddot"
  q_m q_dot_m/1 -> Internal Dynamics/2(q_m q_dot_m)
  f_0/1 -> Euler Poincare/3(f_0)
  Euler Poincare/1(P_dot) -> P_dot/1  "P_dot"
  V/1 -> Euler Poincare/2(V)
  P/1 -> Euler Poincare/1(P)

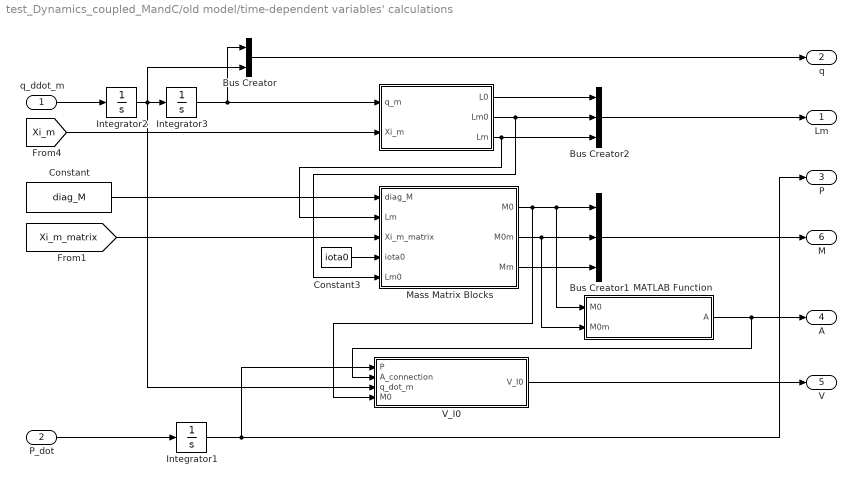
== system test_Dynamics_coupled_MandC/old model/time-dependent variables' calculations ==
  q_ddot_m : Inport
  P_dot : Inport  Port=2
  " " : MATLAB Function  TreatAsAtomicUnit=on
  Bus Creator : BusCreator  Inputs=2
  Bus Creator1 : BusCreator  Inputs=3
  Bus Creator2 : BusCreator  Inputs=3
  Constant : Constant  Value=diag_M  VectorParams1D=off
  Constant3 : Constant  Value=iota0  VectorParams1D=off
  Integrator1 : Integrator
  Integrator2 : Integrator
  Integrator3 : Integrator
  MATLAB Function : MATLAB Function  TreatAsAtomicUnit=on
  Mass Matrix Blocks : Subsystem
  V_I0 : MATLAB Function  TreatAsAtomicUnit=on
  Lm : Outport
  q : Outport  Port=2
  P : Outport  Port=3
  A : Outport  Port=4
  V : Outport  Port=5
  M : Outport  Port=6
  wires:
  Integrator2/1 -> V_I0/3(q_dot_m), Bus Creator/2, Integrator3/1
  q_ddot_m/1 -> Integrator2/1
  " "/1(L0) -> Bus Creator2/1
  " "/3(Lm) -> Mass Matrix Blocks/2(Lm), Bus Creator2/3
  " "/2(Lm0) -> Mass Matrix Blocks/5(Lm0), Bus Creator2/2
  Constant/1 -> Mass Matrix Blocks/1(diag_M)
  [Xi_m_matrix] -> Mass Matrix Blocks/3(Xi_m_matrix)
  [Xi_m] -> " "/2(Xi_m)
  Integrator3/1 -> Bus Creator/1, " "/1(q_m)
  Bus Creator/1 -> q/1
  Mass Matrix Blocks/1(M0) -> V_I0/4(M0), MATLAB Function/1(M0), Bus Creator1/1
  Mass Matrix Blocks/3(Mm) -> Bus Creator1/3
  Bus Creator1/1 -> M/1
  Mass Matrix Blocks/2(M0m) -> MATLAB Function/2(M0m), Bus Creator1/2
  MATLAB Function/1(A) -> V_I0/2(A_connection), A/1
  Constant3/1 -> Mass Matrix Blocks/4(iota0)
  Bus Creator2/1 -> Lm/1
  Integrator1/1 -> V_I0/1(P), P/1
  P_dot/1 -> Integrator1/1
  V_I0/1(V_I0) -> V/1

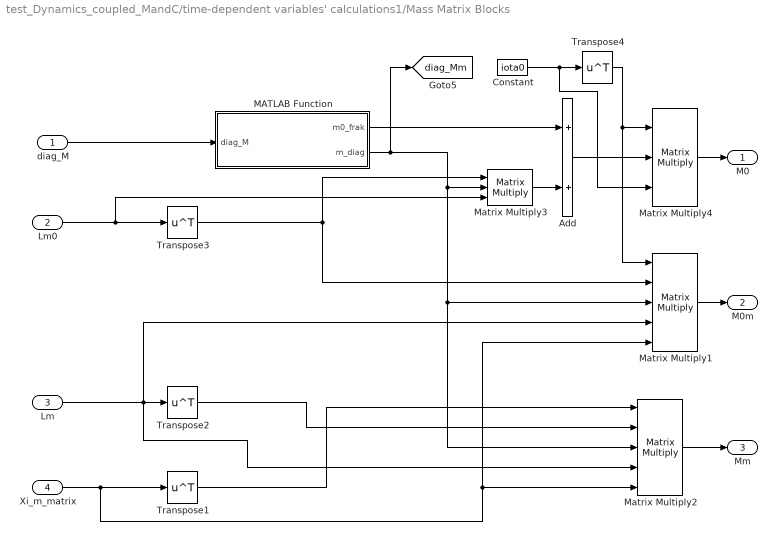
== system test_Dynamics_coupled_MandC/time-dependent variables' calculations1/Mass Matrix Blocks ==
  diag_M : Inport
  Lm0 : Inport  Port=2
  Lm : Inport  Port=3
  Xi_m_matrix : Inport  Port=4
  Add : Sum
  Constant : Constant  Value=iota0
  MATLAB Function : MATLAB Function  TreatAsAtomicUnit=on
  Matrix Multiply1 : Product  Inputs=5  Multiplication=Matrix(*)
  Matrix Multiply2 : Product  Inputs=5  Multiplication=Matrix(*)
  Matrix Multiply3 : Product  Inputs=3  Multiplication=Matrix(*)
  Matrix Multiply4 : Product  Inputs=3  Multiplication=Matrix(*)
  Transpose{1..4} (4 alike) : Math  Operator=transpose  SaturateOnIntegerOverflow=on
  M0 : Outport
  M0m : Outport  Port=2
  Mm : Outport  Port=3
  tag scope: diag_Mm=global
  wires:
  Matrix Multiply2/1 -> Mm/1
  Xi_m_matrix/1 -> Matrix Multiply1/5, Matrix Multiply2/5, Transpose1/1
  diag_M/1 -> MATLAB Function/1(diag_M)
  Lm/1 -> Matrix Multiply1/4, Matrix Multiply2/4, Transpose2/1
  Transpose1/1 -> Matrix Multiply2/1
  Transpose2/1 -> Matrix Multiply2/2
  MATLAB Function/1(m0_frak) -> Add/1
  MATLAB Function/2(m_diag) -> Matrix Multiply3/2, Matrix Multiply2/3, Matrix Multiply1/3, [diag_Mm]
  Matrix Multiply1/1 -> M0m/1
  Add/1 -> Matrix Multiply4/2
  Matrix Multiply3/1 -> Add/2
  Lm0/1 -> Transpose3/1, Matrix Multiply3/3
  Transpose3/1 -> Matrix Multiply3/1, Matrix Multiply1/2
  Constant/1 -> Matrix Multiply4/3, Transpose4/1
  Transpose4/1 -> Matrix Multiply1/1, Matrix Multiply4/1
  Matrix Multiply4/1 -> M0/1

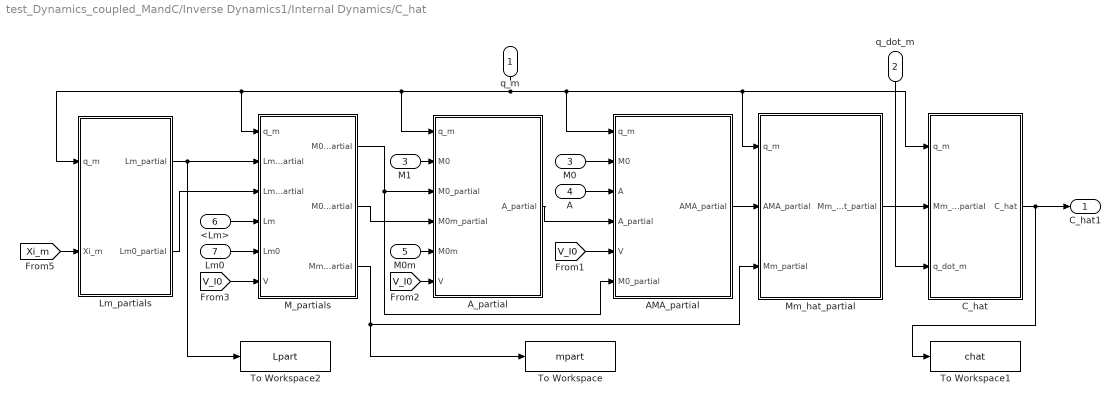
== system test_Dynamics_coupled_MandC/Inverse Dynamics1/Internal Dynamics/C_hat ==
  q_m : Inport
  q_dot_m : Inport  Port=2
  M0 : Inport  Port=3
  A : Inport  Port=4
  M0m : Inport  Port=5
  <Lm> : Inport  Port=6
  Lm0 : Inport  Port=7
  AMA_partial : MATLAB Function  TreatAsAtomicUnit=on
  A_partial : MATLAB Function  TreatAsAtomicUnit=on
  C_hat : MATLAB Function  TreatAsAtomicUnit=on
  Lm_partials : Subsystem
  M1 : InportShadow  Port=3
  M_partials : Subsystem
  Mm_hat_partial : MATLAB Function  TreatAsAtomicUnit=on
  To Workspace : ToWorkspace  VariableName=mpart  SaveFormat=Timeseries  SampleTime=-1
  To Workspace1 : ToWorkspace  VariableName=chat  SaveFormat=Timeseries  SampleTime=-1
  To Workspace2 : ToWorkspace  VariableName=Lpart  SaveFormat=Timeseries  SampleTime=-1
  C_hat1 : Outport
  wires:
  C_hat/1(C_hat) -> To Workspace1/1, C_hat1/1
  q_m/1 -> AMA_partial/1(q_m), Mm_hat_partial/1(q_m), C_hat/1(q_m), A_partial/1(q_m), Lm_partials/1(q_m), M_partials/1(q_m)
  q_dot_m/1 -> C_hat/3(q_dot_m)
  <Lm>/1 -> M_partials/4(Lm)
  [Xi_m] -> Lm_partials/2(Xi_m)
  Lm_partials/1(Lm_partial) -> To Workspace2/1, M_partials/2(Lm_partial)
  M_partials/3(Mm_partial) -> Mm_hat_partial/3(Mm_partial), To Workspace/1
  Mm_hat_partial/1(Mm_hat_partial) -> C_hat/2(Mm_hat_partial)
  AMA_partial/1(AMA_partial) -> Mm_hat_partial/2(AMA_partial)
  M0/1 -> AMA_partial/2(M0)
  M_partials/1(M0_partial) -> A_partial/3(M0_partial), AMA_partial/6(M0_partial)
  A/1 -> AMA_partial/3(A)
  A_partial/1(A_partial) -> AMA_partial/4(A_partial)
  [V_I0] -> AMA_partial/5(V)
  M1/1 -> A_partial/2(M0)
  M0m/1 -> A_partial/5(M0m)
  [V_I0] -> A_partial/6(V)
  M_partials/2(M0m_partial) -> A_partial/4(M0m_partial)
  Lm_partials/2(Lm0_partial) -> M_partials/3(Lm0_partial)
  Lm0/1 -> M_partials/5(Lm0)
  [V_I0] -> M_partials/6(V)

== system test_Dynamics_coupled_MandC/old model/Inverse Dynamics/Euler Poincare ==
  P : Inport
  V : Inport  Port=2
  f_0 : Inport  Port=3
  Add : Sum  Inputs=+-
  Constant : Constant  Value=iota0
  MATLAB Function : MATLAB Function  TreatAsAtomicUnit=on
  Matrix Multiply : Product  Multiplication=Matrix(*)
  To Workspace : ToWorkspace  VariableName=simout  SaveFormat=Timeseries  SampleTime=-1
  Transpose : Math  Operator=transpose  SaturateOnIntegerOverflow=on
  P_dot : Outport
  wires:
  P/1 -> Matrix Multiply/2
  MATLAB Function/1(adj_low) -> Transpose/1
  V/1 -> MATLAB Function/1(V)
  Transpose/1 -> To Workspace/1, Matrix Multiply/1
  Matrix Multiply/1 -> Add/1
  f_0/1 -> Add/2
  Add/1 -> P_dot/1
  Constant/1 -> MATLAB Function/2(iota0)

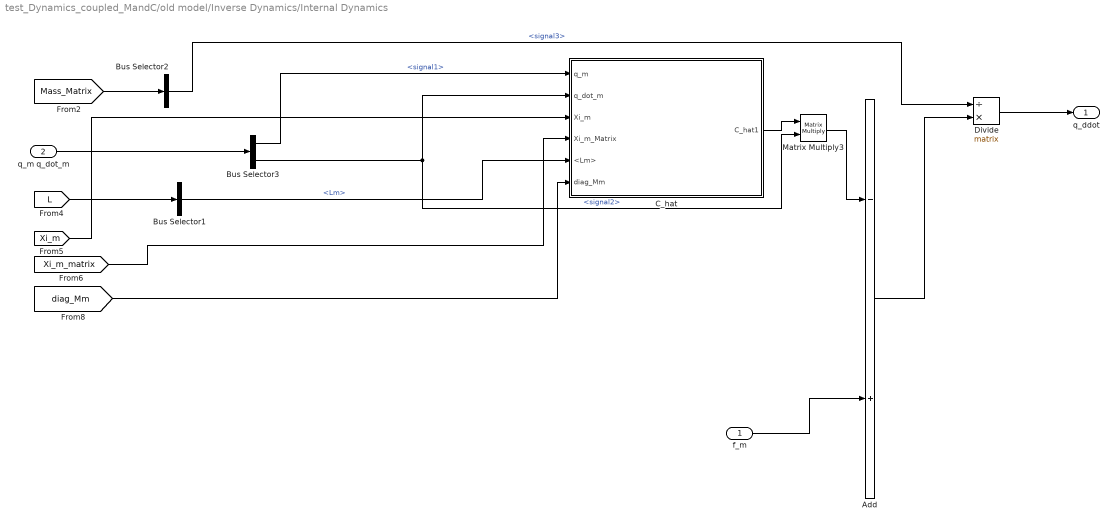
== system test_Dynamics_coupled_MandC/old model/Inverse Dynamics/Internal Dynamics ==
  f_m : Inport
  q_m q_dot_m : Inport  Port=2
  Add : Sum  Inputs=-+
  Bus Selector1 : BusSelector  OutputSignals=Lm
  Bus Selector2 : BusSelector  OutputSignals=signal3
  Bus Selector3 : BusSelector  OutputSignals=signal1,signal2
  C_hat : Subsystem
  Divide : Product  Inputs=/*  Multiplication=Matrix(*)
  Matrix Multiply3 : Product  Multiplication=Matrix(*)
  q_ddot : Outport
  wires:
  f_m/1 -> Add/2
  Divide/1 -> q_ddot/1
  q_m q_dot_m/1 -> Bus Selector3/1
  [Mass_Matrix] -> Bus Selector2/1
  [L] -> Bus Selector1/1
  [Xi_m] -> C_hat/3(Xi_m)
  [Xi_m_matrix] -> C_hat/4(Xi_m_Matrix)
  [diag_Mm] -> C_hat/6(diag_Mm)
  C_hat/1(C_hat1) -> Matrix Multiply3/1
  Matrix Multiply3/1 -> Add/1
  Add/1 -> Divide/2
  Bus Selector3/2 -> Matrix Multiply3/2, C_hat/2(q_dot_m)  "<signal2>"
  Bus Selector3/1 -> C_hat/1(q_m)  "<signal1>"
  Bus Selector1/1 -> C_hat/5(<Lm>)  "<Lm>"
  Bus Selector2/1 -> Divide/1  "<signal3>"

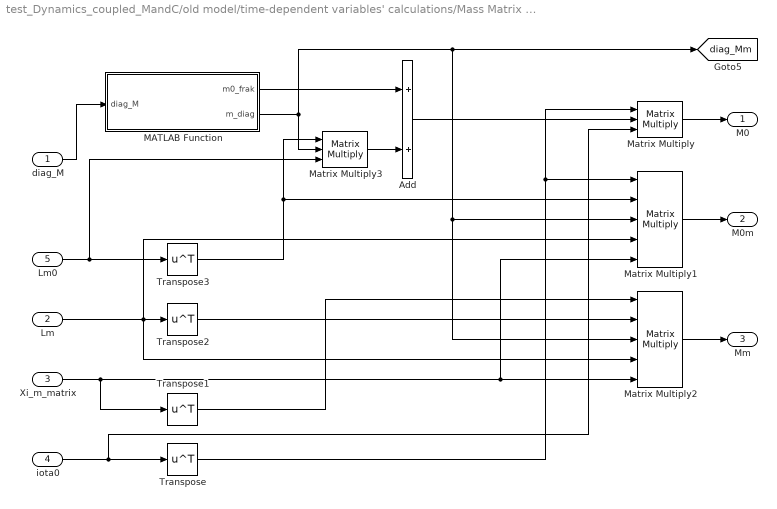
== system test_Dynamics_coupled_MandC/old model/time-dependent variables' calculations/Mass Matrix Blocks ==
  diag_M : Inport
  Lm : Inport  Port=2
  Xi_m_matrix : Inport  Port=3
  iota0 : Inport  Port=4
  Lm0 : Inport  Port=5
  Add : Sum
  MATLAB Function : MATLAB Function  TreatAsAtomicUnit=on
  Matrix Multiply : Product  Inputs=3  Multiplication=Matrix(*)
  Matrix Multiply1 : Product  Inputs=5  Multiplication=Matrix(*)
  Matrix Multiply2 : Product  Inputs=5  Multiplication=Matrix(*)
  Matrix Multiply3 : Product  Inputs=3  Multiplication=Matrix(*)
  Transpose{,1..3} (4 alike) : Math  Operator=transpose  SaturateOnIntegerOverflow=on
  M0 : Outport
  M0m : Outport  Port=2
  Mm : Outport  Port=3
  tag scope: diag_Mm=global
  wires:
  Matrix Multiply2/1 -> Mm/1
  Xi_m_matrix/1 -> Transpose1/1, Matrix Multiply1/5, Matrix Multiply2/5
  diag_M/1 -> MATLAB Function/1(diag_M)
  Lm/1 -> Matrix Multiply2/4, Matrix Multiply1/4, Transpose2/1
  Transpose1/1 -> Matrix Multiply2/1
  Transpose2/1 -> Matrix Multiply2/2
  MATLAB Function/2(m_diag) -> Matrix Multiply1/3, Matrix Multiply2/3, [diag_Mm], Matrix Multiply3/2
  Matrix Multiply1/1 -> M0m/1
  Matrix Multiply/1 -> M0/1
  iota0/1 -> Matrix Multiply/3, Transpose/1
  Transpose/1 -> Matrix Multiply/1, Matrix Multiply1/1
  Add/1 -> Matrix Multiply/2
  Matrix Multiply3/1 -> Add/2
  MATLAB Function/1(m0_frak) -> Add/1
  Lm0/1 -> Matrix Multiply3/3, Transpose3/1
  Transpose3/1 -> Matrix Multiply1/2, Matrix Multiply3/1

== system test_Dynamics_coupled_MandC/Inverse Dynamics1/Internal Dynamics/C_hat/Lm_partials ==
  q_m : Inport
  Xi_m : Inport  Port=2
  Constant : Constant  Value=iota0
  Lm0partial : MATLAB Function  TreatAsAtomicUnit=on
  Lmpartial : MATLAB Function  TreatAsAtomicUnit=on
  Lm_partial : Outport
  Lm0_partial : Outport  Port=2
  wires:
  Lmpartial/1(Lm_partial) -> Lm_partial/1
  Lm0partial/1(Lm0_partial) -> Lm0_partial/1
  Constant/1 -> Lm0partial/3(iota0), Lmpartial/3(iota0)
  q_m/1 -> Lm0partial/1(q_m), Lmpartial/1(q_m)
  Xi_m/1 -> Lm0partial/2(Xi_m), Lmpartial/2(Xi_m)

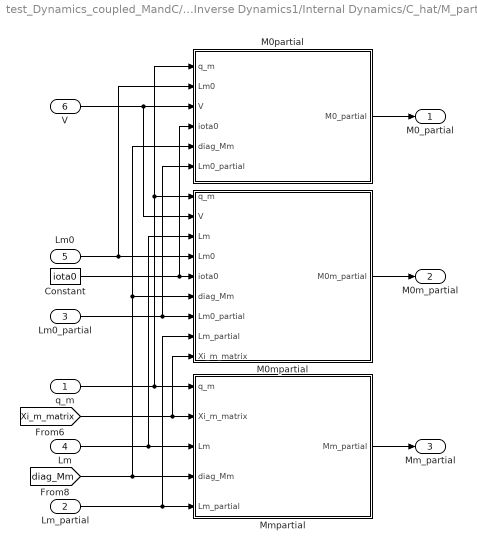
== system test_Dynamics_coupled_MandC/Inverse Dynamics1/Internal Dynamics/C_hat/M_partials ==
  q_m : Inport
  Lm_partial : Inport  Port=2
  Lm0_partial : Inport  Port=3
  Lm : Inport  Port=4
  Lm0 : Inport  Port=5
  V : Inport  Port=6
  " M0partial" : MATLAB Function  TreatAsAtomicUnit=on
  Constant : Constant  Value=iota0
  M0mpartial : MATLAB Function  TreatAsAtomicUnit=on
  Mmpartial : MATLAB Function  TreatAsAtomicUnit=on
  M0_partial : Outport
  M0m_partial : Outport  Port=2
  Mm_partial : Outport  Port=3
  wires:
  Lm_partial/1 -> M0mpartial/8(Lm_partial), Mmpartial/5(Lm_partial)
  q_m/1 -> " M0partial"/1(q_m), M0mpartial/1(q_m), Mmpartial/1(q_m)
  [diag_Mm] -> " M0partial"/5(diag_Mm), M0mpartial/6(diag_Mm), Mmpartial/4(diag_Mm)
  [Xi_m_matrix] -> M0mpartial/9(Xi_m_matrix), Mmpartial/2(Xi_m_matrix)
  Lm/1 -> M0mpartial/3(Lm), Mmpartial/3(Lm)
  Mmpartial/1(Mm_partial) -> Mm_partial/1
  M0mpartial/1(M0m_partial) -> M0m_partial/1
  " M0partial"/1(M0_partial) -> M0_partial/1
  Lm0/1 -> " M0partial"/2(Lm0), M0mpartial/4(Lm0)
  Lm0_partial/1 -> " M0partial"/6(Lm0_partial), M0mpartial/7(Lm0_partial)
  Constant/1 -> " M0partial"/4(iota0), M0mpartial/5(iota0)
  V/1 -> M0mpartial/2(V), " M0partial"/3(V)

== system test_Dynamics_coupled_MandC/old model/Inverse Dynamics/Internal Dynamics/C_hat ==
  q_m : Inport
  q_dot_m : Inport  Port=2
  Xi_m : Inport  Port=3
  Xi_m_Matrix : Inport  Port=4
  <Lm> : Inport  Port=5
  diag_Mm : Inport  Port=6
  C_hat : MATLAB Function  TreatAsAtomicUnit=on
  Lm_partials : Subsystem
  M_partials : Subsystem
  C_hat1 : Outport
  wires:
  C_hat/1(C_hat) -> C_hat1/1
  q_m/1 -> C_hat/1(q_m), M_partials/1(q_m), Lm_partials/1(q_m)
  q_dot_m/1 -> C_hat/2(q_dot_m)
  Xi_m_Matrix/1 -> M_partials/3(Xi_m_Matrix)
  <Lm>/1 -> M_partials/4(Lm)
  diag_Mm/1 -> M_partials/5(diag_Mm)
  Xi_m/1 -> Lm_partials/2(Xi_m)
  Lm_partials/1(Lm_partial) -> M_partials/2(Lm_partial)
  M_partials/1(Mm_partial) -> C_hat/3(Mm_hat_partial)

== system test_Dynamics_coupled_MandC/old model/Inverse Dynamics/Internal Dynamics/C_hat/Lm_partials ==
  q_m : Inport
  Xi_m : Inport  Port=2
  Constant : Constant  Value=iota0
  Lmpartial : MATLAB Function  TreatAsAtomicUnit=on
  Lm_partial : Outport
  wires:
  Xi_m/1 -> Lmpartial/2(Xi_m)
  q_m/1 -> Lmpartial/1(q_m)
  Lmpartial/1(Lm_partial) -> Lm_partial/1
  Constant/1 -> Lmpartial/3(iota0)

== system test_Dynamics_coupled_MandC/old model/Inverse Dynamics/Internal Dynamics/C_hat/M_partials ==
  q_m : Inport
  Lm_partial : Inport  Port=2
  Xi_m_Matrix : Inport  Port=3
  Lm : Inport  Port=4
  diag_Mm : Inport  Port=5
  Mmpartial : MATLAB Function  TreatAsAtomicUnit=on
  Mm_partial : Outport
  wires:
  Lm_partial/1 -> Mmpartial/5(Lm_partial)
  q_m/1 -> Mmpartial/1(q_m)
  diag_Mm/1 -> Mmpartial/4(diag_Mm)
  Xi_m_Matrix/1 -> Mmpartial/2(Xi_m_Matrix)
  Lm/1 -> Mmpartial/3(Lm)
  Mmpartial/1(Mm_partial) -> Mm_partial/1

== matlab function test_Dynamics_coupled_MandC/old model/Inverse Dynamics/Euler Poincare/MATLAB Function ==
  data: V input; adj_low output; iota0 input
function adj_low = adj_low(V, iota0)
% calculates the adjoint corresponding to the Lie bracket of vector V and ()
adj_low = adjoint_low(V,iota0);

== matlab function test_Dynamics_coupled_MandC/old model/Inverse Dynamics/Internal Dynamics/C_hat/C_hat ==
  data: q_m input; q_dot_m input; C_hat output; Mm_hat_partial input
function C_hat = C_hat(q_m,q_dot_m, Mm_hat_partial)
% Calculates the C_hat_m matrix from base pose and arm joint angles

n=length(q_m);


% Calculate C_hat matrix
C_temp1=zeros(n,n);
C_temp2=zeros(n,n);
C_hat=zeros(n,n);
for i=1:n
    C_temp1=C_temp1+Mm_hat_partial(1:n,1:n,i).*q_dot_m(i); % nxn by scalar
    C_temp2(i,1:n)=0.5*transpose(q_dot_m)*Mm_hat_partial(1:n,1:n,i); %1xn by nxn 
end

C_hat=C_temp1-C_temp2;

== matlab function test_Dynamics_coupled_MandC/Inverse Dynamics1/Internal Dynamics/C_hat/Lm_partials/Lm0partial ==
  data: q_m input; Lm0_partial output; Xi_m input; iota0 input
function Lm0_partial = Lm0_partial(q_m,Xi_m,iota0)
% Calculates the C_hat_m matrix from base pose and arm joint angles

n=length(q_m);

% Find partial of Lm to joint angles
Lm0_partial=zeros(6*n,6,n); % 6nx6xn
for i=1:n
    for j=1:n
        Lm0_partial(6*(j-1)+1:6*j,1:6,i)=Ad_partial(j,1,i,Xi_m,q_m,iota0); % equation 114 of TRO paper
    end
end

%%%%%%%%%%%%%%%%%%%%%%%%%%%%%%%%%%%%%%%%%%%%%%%%%%%%%%%%%%%%% MUST BE
%%%%%%%%%%%%%%%%%%%%%%%%%%%%%%%%%%%%%%%%%%%%%%%%%%%%%%%%%%%%% CHECKED

== matlab function test_Dynamics_coupled_MandC/Inverse Dynamics1/Internal Dynamics/M_hat ==
  data: M0 input; Mm input; A input; M_hat output
function M_hat =M_hat(M0,Mm,A)
% Compute the Mass Matrix of the multibody system.
%   Input:
%   M0      Spacecraft mass matrix 
%   M0m     Coupling
%   Mm      Manipulator mass matrix

% Calculate M_hat
M_hat=Mm-transpose(A)*M0*A;


end

== matlab function test_Dynamics_coupled_MandC/old model/time-dependent variables' calculations/  ==
  data: q_m input; L0 output; Lm0 output; Lm output; Xi_m input
function [L0,Lm0,Lm] =L_calculator(q_m,Xi_m)
% Calculates the time-dependent L matrix
n=length(q_m);
L=zeros(6*(n+1),6*(n+1));
% Compute M_frak for ith body
% Calculate L matrix
for i=1:n+1
    for j=1:n+1
        if i>j
            Ad_temp=eye(6);
            for k=j:i-1
                Ad_temp=Adjoint(g_Matrix(-Xi_m(:,k),q_m(k)))*Ad_temp;
            end
            L(6*(i-1)+1:6*(i-1)+6,6*(j-1)+1:6*(j-1)+6)=Ad_temp;
        elseif i==j
            L(6*(i-1)+1:6*(i-1)+6,6*(j-1)+1:6*(j-1)+6)=eye(6);
        elseif i<j
            L(6*(i-1)+1:6*(i-1)+6,6*(j-1)+1:6*(j-1)+6)=zeros(6);
        end
    end
end

L0=L(1:6,1:6);
Lm0=L(7:end,1:6);
Lm=L(7:end,7:end);

end

== matlab function test_Dynamics_coupled_MandC/time-dependent variables' calculations1/MATLAB Function ==
  data: M0 input; M0m input; A output
function A=A_connection(M0,M0m)
% Compute the connection A from mass properties

A=M0\M0m;

== matlab function test_Dynamics_coupled_MandC/old model/Inverse Dynamics/Internal Dynamics/C_hat/Lm_partials/Lmpartial ==
  data: q_m input; Lm_partial output; Xi_m input; iota0 input
function Lm_partial  = Lm_partial(q_m,Xi_m,iota0)
% Calculates the C_hat_m matrix from base pose and arm joint angles

n=length(q_m);

% Find partial of Lm0 to joint angles
Lm_partial=zeros(6*n,6*n,n); % 6nx6xn
for i=1:n
    for j=1:n
        for k=1:n
            if j==k
                Lm_partial(6*(j-1)+1:6*(j-1)+6,6*(k-1)+1:6*(k-1)+6,i)=eye(6,6);
            elseif j>i && i>=k
                Lm_partial(6*(j-1)+1:6*j,6*(k-1)+1:6*k,i)=-Ad_frak(j,i+1,Xi_m,q_m)*adjoint_low(Xi_m(:,i),iota0)*Ad_frak(i,k,Xi_m,q_m); % equation 81 of TRO paper
            elseif i==j && i>=k
                Lm_partial(6*(j-1)+1:6*j,6*(k-1)+1:6*k,i)=-adjoint_low(Xi_m(:,i),iota0)*Ad_frak(i,k,Xi_m,q_m); % equation 81 of TRO paper
            else
                Lm_partial(6*(j-1)+1:6*(j-1)+6,6*(k-1)+1:6*(k-1)+6,i)=zeros(6,6);
            end

        end
    end
end

== matlab function test_Dynamics_coupled_MandC/Inverse Dynamics1/Internal Dynamics/C_hat/M_partials/ M0partial ==
  data: q_m input; M0_partial output; Lm0 input; V input; iota0 input; diag_Mm input; Lm0_partial input
function M0_partial = M0_partial(q_m,Lm0,V,iota0,diag_Mm,Lm0_partial)
% Calculates the C_hat_m matrix from base pose and arm joint angles

n=length(q_m);
b=length(V);

% Find partial of M0 to joint angles
M0_partial=zeros(b,b,n); %initiate
for i=1:n
    M0_partial(1:b,1:b,i)= iota0'*(transpose(Lm0_partial(1:end,1:end,i))*diag_Mm*Lm0+transpose(Lm0)*diag_Mm*Lm0_partial(1:end,1:end,i))*iota0; %6x6 %equation 117 of TRO
end
